simulink model "adrc"  (R2021a)
settings: Solver=FixedStepAuto  StartTime=0.0  StopTime=20  FixedStep=0.0025  RelTol=1e-3
libraries: pid_lib x1
settings Model: Creator=liuya  LastModifiedBy=liuya

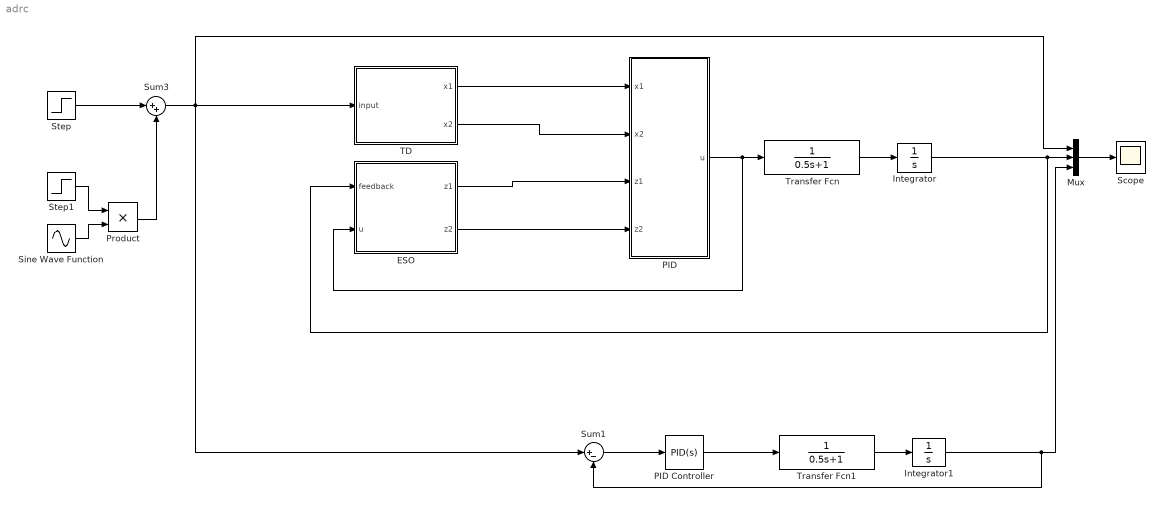
== system adrc ==
  ESO : Subsystem
  Integrator : Integrator
  Integrator1 : Integrator
  Mux : Mux  Inputs=3
  PID : Subsystem
  PID Controller : pid_lib/PID Controller  Controller=PID  Form=Parallel  TimeDomain=Continuous-time  UseExternalTs=off  SampleTime=-1  IntegratorMethod=Forward Euler  FilterMethod=Forward Euler  ControllerParametersSource=internal  P=8  I=0  D=4  UseFilter=on  N=100  TunerSelectOption=Transfer Function Based (PID Tuner App)  InitialConditionSource=internal  InitialConditionForIntegrator=0  InitialConditionForFilter=0  DifferentiatorICPrevScaledInput=0  ExternalReset=none  TrackingMode=off  Kt=1  LimitOutput=off  SatLimitsSource=internal  UpperSaturationLimit=inf  LowerSaturationLimit=-inf  LinearizeAsGain=on  AntiWindupMode=none  Kb=1  POutMin=[]  POutMax=[]  IOutMin=[]  IOutMax=[]  DOutMin=[]  DOutMax=[]  NOutMin=[]  NOutMax=[]  SumOutMin=[]  SumOutMax=[]  SaturationOutMin=[]  SaturationOutMax=[]  PParamMin=[]  PParamMax=[]  IParamMin=[]  IParamMax=[]  DParamMin=[]  DParamMax=[]  NParamMin=[]  NParamMax=[]  KbParamMin=[]  KbParamMax=[]  KtParamMin=[]  KtParamMax=[]  KbOutMin=[]  KbOutMax=[]  KtOutMin=[]  KtOutMax=[]  IntegratorOutMin=[]  IntegratorOutMax=[]  FilterOutMin=[]  FilterOutMax=[]  SumI1OutMin=[]  SumI1OutMax=[]  SumI2OutMin=[]  SumI2OutMax=[]  SumI3OutMin=[]  SumI3OutMax=[]  SumI4OutMin=[]  SumI4OutMax=[]  SumDOutMin=[]  SumDOutMax=[]  DifferentiatorOutMin=[]  DifferentiatorOutMax=[]  FilterDiffOutCoefMin=[]  FilterDiffOutCoefMax=[]  ReciprocalOutMin=[]  ReciprocalOutMax=[]  SumDenOutMin=[]  SumDenOutMax=[]  SumNumOutMin=[]  SumNumOutMax=[]  DivideOutMin=[]  DivideOutMax=[]  UdiffTsProdOutMin=[]  UdiffTsProdOutMax=[]  NTsProdOutMin=[]  NTsProdOutMax=[]  UintegralTsProdOutMin=[]  UintegralTsProdOutMax=[]  UngainTsProdOutMin=[]  UngainTsProdOutMax=[]  IntegratorContinuousStateAttributes=''  IntegratorStateMustResolveToSignalObject=off  IntegratorRTWStateStorageClass=Auto  FilterContinuousStateAttributes=''  FilterStateMustResolveToSignalObject=off  FilterRTWStateStorageClass=Auto  ParallelPVariant=InternalParameters  IdealPVariant=Disabled  IVariant=InternalParameters  DVariant=InternalParameters  IntegratorVariant=Continuous  SatVariant=Disabled  AWVariant=Passthrough  PCopyVariant=Disabled  TRVariant=Disabled  FdbkBlocksVariant=Forward  IdealPFdbkVariant=Disabled  SatFdbkVariant=Disabled  DerivativeFilterVariant=ContFilter  NVariant=InternalParameters  NCopyVariant=Disabled  FilterICVariant=InternalICsFilter  IntegratorICVariant=InternalICs  ExternalResetVariant=Disabled  TRSumVariant=Passthrough  SumFdbkVariant=Disabled  SumVariant=Sum_PID  TsampFilterVariant=InternalTs  TsampNgainVariant=Passthrough  TsampIntegralVariant=Passthrough  ExternalSaturationOutDataTypeStr=Inherit: Same as second input
  Product : Product
  Scope : Scope
  Sine Wave Function : Sin  Frequency=2 * 3.1415926  SampleTime=0
  Step : Step  After=10  SampleTime=0
  Step1 : Step  Time=5  SampleTime=0
  Sum1 : Sum  Inputs=|+-
  Sum3 : Sum  Inputs=|++
  TD : Subsystem
  Transfer Fcn : TransferFcn  Denominator=[0.5 1]
  Transfer Fcn1 : TransferFcn  Denominator=[0.5 1]
  wires:
  Sum3/1 -> Mux/1, Sum1/1, TD/1(input)
  TD/1(x1) -> PID/1(x1)
  PID/1(u) -> Transfer Fcn/1, ESO/2(u)
  Mux/1 -> Scope/1
  TD/2(x2) -> PID/2(x2)
  ESO/2(z2) -> PID/4(z2)
  ESO/1(z1) -> PID/3(z1)
  Transfer Fcn/1 -> Integrator/1
  Integrator/1 -> ESO/1(feedback), Mux/2
  PID Controller/1 -> Transfer Fcn1/1
  Transfer Fcn1/1 -> Integrator1/1
  Sum1/1 -> PID Controller/1
  Integrator1/1 -> Sum1/2, Mux/3
  Step/1 -> Sum3/1
  Step1/1 -> Product/1
  Sine Wave Function/1 -> Product/2
  Product/1 -> Sum3/2

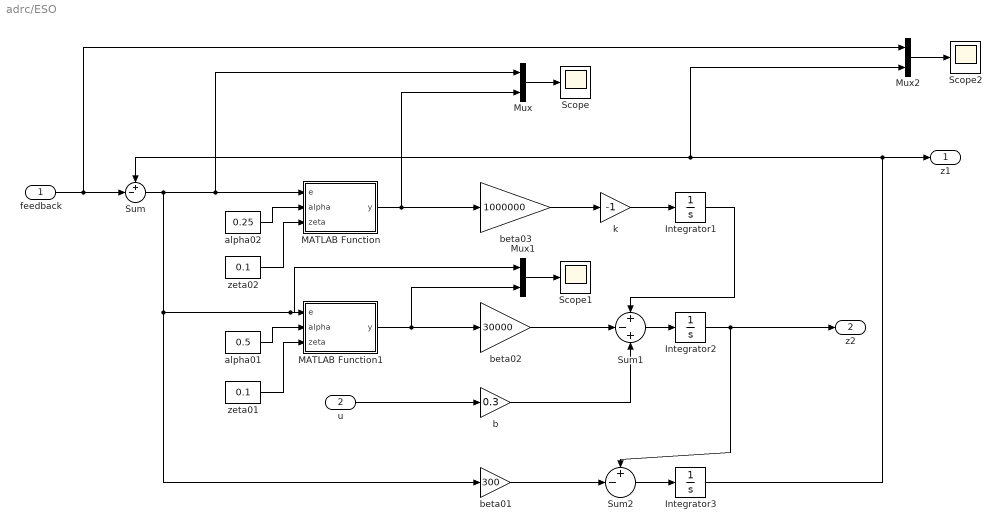
== system adrc/ESO ==
  feedback : Inport
  u : Inport  Port=2
  Integrator1 : Integrator
  Integrator2 : Integrator
  Integrator3 : Integrator
  MATLAB Function : MATLAB Function  TreatAsAtomicUnit=on
  MATLAB Function1 : MATLAB Function  TreatAsAtomicUnit=on
  Mux : Mux  Inputs=2
  Mux1 : Mux  Inputs=2
  Mux2 : Mux  Inputs=2
  Scope : Scope
  Scope1 : Scope
  Scope2 : Scope
  Sum : Sum  Inputs=+-|
  Sum1 : Sum  Inputs=+-+
  Sum2 : Sum  Inputs=+-|
  alpha01 : Constant  Value=0.5
  alpha02 : Constant  Value=0.25
  b : Gain  Gain=0.3
  beta01 : Gain  Gain=300
  beta02 : Gain  Gain=30000
  beta03 : Gain  Gain=1000000
  k : Gain  Gain=-1
  zeta01 : Constant  Value=0.1
  zeta02 : Constant  Value=0.1
  z1 : Outport
  z2 : Outport  Port=2
  wires:
  Integrator2/1 -> z2/1, Sum2/1
  b/1 -> Sum1/3
  alpha01/1 -> MATLAB Function1/2(alpha)
  beta02/1 -> Sum1/2
  Sum2/1 -> Integrator3/1
  MATLAB Function/1(y) -> Mux/2, beta03/1
  Integrator1/1 -> Sum1/1
  beta01/1 -> Sum2/2
  u/1 -> b/1
  alpha02/1 -> MATLAB Function/2(alpha)
  beta03/1 -> k/1
  zeta01/1 -> MATLAB Function1/3(zeta)
  zeta02/1 -> MATLAB Function/3(zeta)
  Sum1/1 -> Integrator2/1
  Mux/1 -> Scope/1
  k/1 -> Integrator1/1
  Mux1/1 -> Scope1/1
  Sum/1 -> Mux/1, MATLAB Function/1(e), beta01/1, Mux1/1, MATLAB Function1/1(e)
  MATLAB Function1/1(y) -> Mux1/2, beta02/1
  Mux2/1 -> Scope2/1
  feedback/1 -> Mux2/1, Sum/2
  Integrator3/1 -> z1/1, Mux2/2, Sum/1

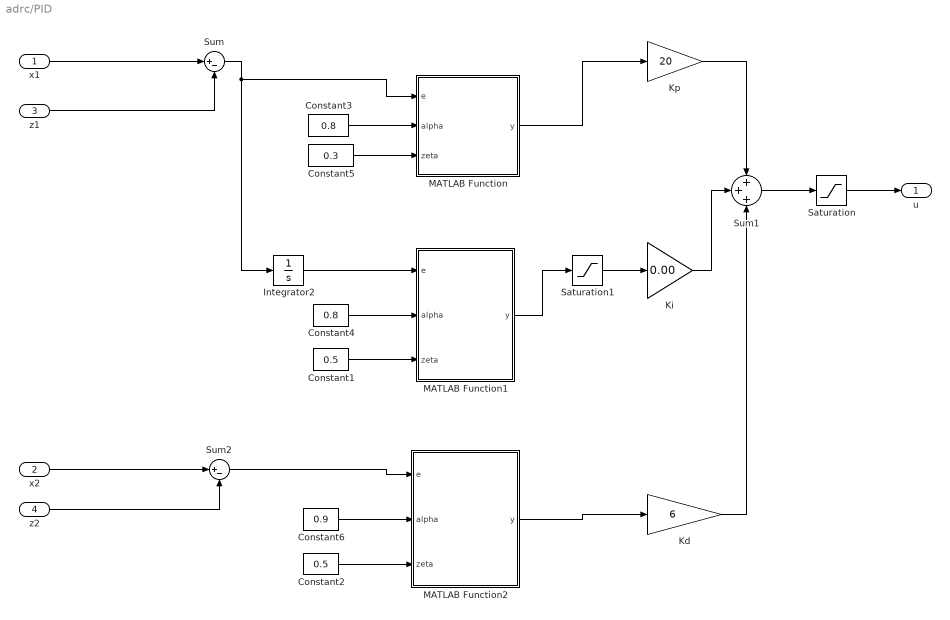
== system adrc/PID ==
  x1 : Inport
  x2 : Inport  Port=2
  z1 : Inport  Port=3
  z2 : Inport  Port=4
  Constant1 : Constant  Value=0.5
  Constant2 : Constant  Value=0.5
  Constant3 : Constant  Value=0.8
  Constant4 : Constant  Value=0.8
  Constant5 : Constant  Value=0.3
  Constant6 : Constant  Value=0.9
  Integrator2 : Integrator
  Kd : Gain  Gain=6
  Ki : Gain  Gain=0.00
  Kp : Gain  Gain=20
  MATLAB Function : MATLAB Function  TreatAsAtomicUnit=on
  MATLAB Function1 : MATLAB Function  TreatAsAtomicUnit=on
  MATLAB Function2 : MATLAB Function  TreatAsAtomicUnit=on
  Saturation : Saturate  UpperLimit=100  LowerLimit=-100
  Saturation1 : Saturate  UpperLimit=50  LowerLimit=-50
  Sum : Sum  Inputs=|+-
  Sum1 : Sum  Inputs=+++
  Sum2 : Sum  Inputs=|+-
  u : Outport
  wires:
  z1/1 -> Sum/2
  Kp/1 -> Sum1/1
  Constant6/1 -> MATLAB Function2/2(alpha)
  Constant4/1 -> MATLAB Function1/2(alpha)
  Constant1/1 -> MATLAB Function1/3(zeta)
  Constant5/1 -> MATLAB Function/3(zeta)
  Kd/1 -> Sum1/3
  z2/1 -> Sum2/2
  Saturation/1 -> u/1
  Constant3/1 -> MATLAB Function/2(alpha)
  Ki/1 -> Sum1/2
  Saturation1/1 -> Ki/1
  Sum1/1 -> Saturation/1
  x2/1 -> Sum2/1
  x1/1 -> Sum/1
  Constant2/1 -> MATLAB Function2/3(zeta)
  MATLAB Function1/1(y) -> Saturation1/1
  Integrator2/1 -> MATLAB Function1/1(e)
  Sum/1 -> MATLAB Function/1(e), Integrator2/1
  MATLAB Function/1(y) -> Kp/1
  MATLAB Function2/1(y) -> Kd/1
  Sum2/1 -> MATLAB Function2/1(e)

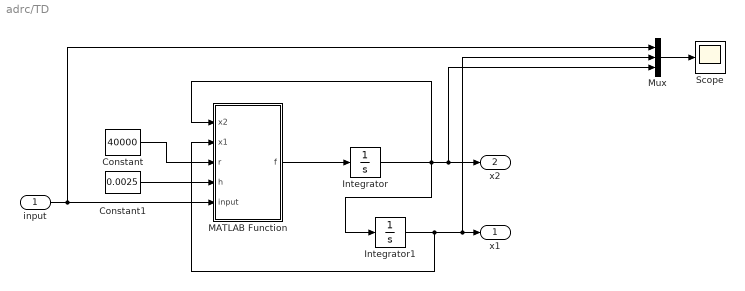
== system adrc/TD ==
  input : Inport
  Constant : Constant  Value=40000
  Constant1 : Constant  Value=0.0025
  Integrator : Integrator
  Integrator1 : Integrator
  MATLAB Function : MATLAB Function  TreatAsAtomicUnit=on
  Mux : Mux  Inputs=3
  Scope : Scope
  x1 : Outport
  x2 : Outport  Port=2
  wires:
  input/1 -> Mux/1, MATLAB Function/5(input)
  Constant/1 -> MATLAB Function/3(r)
  Constant1/1 -> MATLAB Function/4(h)
  MATLAB Function/1(f) -> Integrator/1
  Integrator/1 -> Integrator1/1, MATLAB Function/1(x2), Mux/3, x2/1
  Integrator1/1 -> Mux/2, x1/1, MATLAB Function/2(x1)
  Mux/1 -> Scope/1

== matlab function adrc/ESO/MATLAB Function ==
  data: e input; y output; alpha input; zeta input
function y = fal(e, alpha, zeta)
s = 0.5 * (sign(e + zeta) - sign(e - zeta));
y = (e * s / power(zeta, 1-alpha)) + power(abs(e), alpha) * sign(e) * (1-s);

== matlab function adrc/TD/MATLAB Function ==
  data: x2 input; x1 input; f output; r input; h input; input input
% 二阶最速微分跟踪函数
% x1 为对输入 input 的非线性低通滤波输出，阶跃输入响应为 s 型上升输出
% x2 为对输入 input 的微分估计输出
% r 为调节系数，r越大跟踪快速性越好，但微分信号会增加高频噪声
% h 为调节步长，可取为控制周期 dt 或 dt 的 N 倍，越大对高频噪声的抑制越强，但对应滞后也大
function f=fst(x2,x1,r,h,input)
d=r*h;     
d0=r*h*h;	
y=x1-input+h*x2;
a0=sqrt(d^2+8*r*abs(y));
if abs(y)<=d0
    a=x2+y/h;
else
    a=x2+0.5*(a0-d)*sign(y);
end
if abs(a)<=d
    f=-r*a/d;
else
    f=-r*sign(a);
end

== matlab function adrc/ESO/MATLAB Function1 ==
  data: e input; y output; alpha input; zeta input
function y = fal(e, alpha, zeta)
s = 0.5 * (sign(e + zeta) - sign(e - zeta));
y = (e * s / power(zeta, 1-alpha)) + power(abs(e), alpha) * sign(e) * (1-s);

== matlab function adrc/PID/MATLAB Function ==
  data: e input; y output; alpha input; zeta input
function y = fal(e, alpha, zeta)
s = 0.5 * (sign(e + zeta) - sign(e - zeta));
y = (e * s / power(zeta, 1-alpha)) + power(abs(e), alpha) * sign(e) * (1-s);

== matlab function adrc/PID/MATLAB Function1 ==
  data: e input; y output; alpha input; zeta input
% 非线性处理函数，当 alpha 小于 1 时，输出 y 以 zeta 为门限，超过 zeta 的 e 会被衰减，小于 zeta 的 e 会被增强
% 当 alpha 大于 1 时则相反，超过 zeta 的 e 会被增强，小于 zeta 的 e 会被衰减
% alpha 偏离 1 越多，则非线性作用越强，若 alhpa 为 1，则 y = e 无非线性调节作用
function y = fal(e, alpha, zeta)

s = 0.5 * (sign(e + zeta) - sign(e - zeta));
y = (e * s / power(zeta, 1-alpha)) + power(abs(e), alpha) * sign(e) * (1-s);

== matlab function adrc/PID/MATLAB Function2 ==
  data: e input; y output; alpha input; zeta input
function y = fal(e, alpha, zeta)
s = 0.5 * (sign(e + zeta) - sign(e - zeta));
y = (e * s / power(zeta, 1-alpha)) + power(abs(e), alpha) * sign(e) * (1-s);
